simulink model "my_PUMA"  (Simulink 10.3)
settings: Solver=ode45  StartTime=0.0  StopTime=5  MaxStep=10  RelTol=1e-3  AbsTol=1e-6
StopFcn:
  | run('End_point_graph.m')
values from neighbouring files (symbols this model uses):
  k_p1 = (w_n1^2).*T_m1 ./ K1    [vars.m]
  k_p2 = (w_n2^2).*T_m2 ./ K2    [vars.m]
  k_p3 = (w_n3^2).*T_m3 ./ K3    [vars.m]
  k_v1 = 2*w_n1*zeta1*T_m1./(K1+1)    [vars.m]
  k_v2 = 2*w_n2*zeta2*T_m2./(K2+1)    [vars.m]
  k_v3 = 2*w_n3*zeta3*T_m3./(K3+1)    [vars.m]
  ng1 = 40+gn*4    [vars.m]
  ng2 = 100-gn*2    [vars.m]
  ng3 = 60+gn    [vars.m]
  thr10 = inital_angles(1)    [vars.m]
  thr20 = inital_angles(2)    [vars.m]
  thr30 = inital_angles(3)    [vars.m]
settings Model: Creator=Gu  LastModifiedBy=mubeen ak  MultithreadedSim=on
settings SolverCC: AutoScaleAbsTol=off
settings DataIOCC: SaveOutput=off  SaveTime=off  SignalLoggingName=sigsOut
settings OptimizationCC: BlockReduction=off  BooleanDataType=off  InitFltsAndDblsToZero=on
settings DebuggingCC: SaveWithParameterizedLinksMsg=none  SignalResolutionControl=TryResolveAllWithWarning  MultiTaskDSMMsg=warning  MultiTaskCondExecSysMsg=none  SFExecutionAtInitializationDiag=warning  SFMachineParentedDataDiag=error
settings HardwareCC: TargetUnknown=on
settings RTWCC: DLArmComputeVersion=20.02.1
settings GRTTargetCC: TargetFcnLib=ansi_tfl_tmw.mat
settings ConfigComp: CovSFcnEnable=off

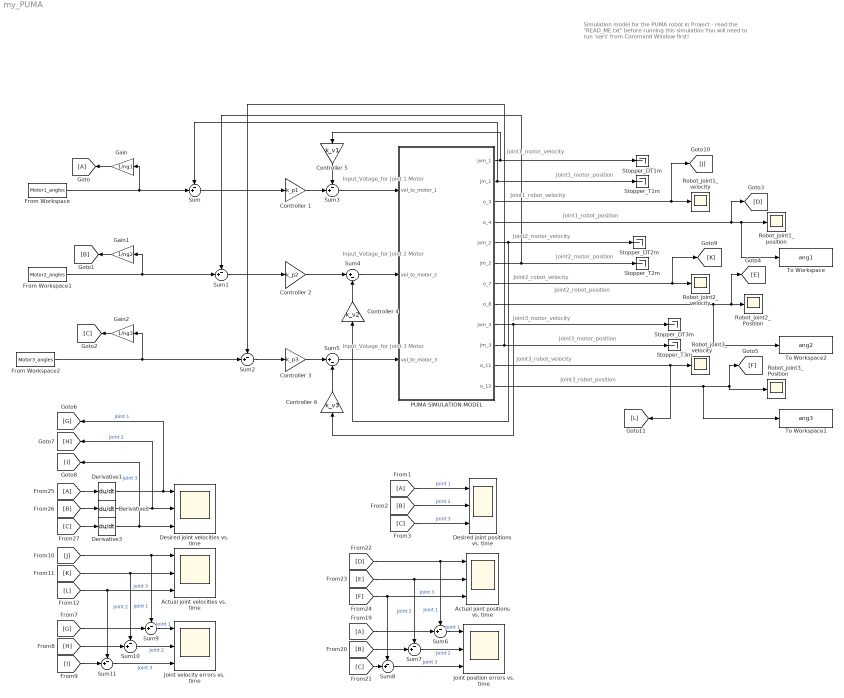
== system my_PUMA ==
  note: Joint1_motor_position
  note: Simulation model for the PUMA robot in Project - read the "READ_ME.txt" before running this simulation
      | You will need to run 'vars' from Command Window first!
  note: Joint2_motor_position
  note: Joint3_motor_position
  note: Joint1_motor_velocity
  note: Joint2_motor_velocity
  note: Joint3_motor_velocity
  note: Joint1_robot_velocity
  note: Joint2_robot_velocity
  note: Joint3_robot_velocity
  note: Joint1_robot_position
  note: Joint2_robot_position
  note: Joint3_robot_position
  note: Input_Votage_for Joint 3 Motor
  note: Input_Votage_for Joint 2 Motor
  note: Input_Votage_for Joint 1 Motor
  "Actual joint positions vs. time " : Scope  NumInputPorts=3
  "Actual joint velocities vs. time " : Scope  NumInputPorts=3
  Controller 1 : Gain  Gain=k_p1
  Controller 2 : Gain  Gain=k_p2
  Controller 3 : Gain  Gain=k_p3
  Controller 4 : Gain  Gain=k_v2
  Controller 5 : Gain  Gain=k_v1
  Controller 6 : Gain  Gain=k_v3
  Derivative1 : Derivative
  Derivative2 : Derivative
  Derivative3 : Derivative
  Desired joint positions vs. time : Scope  NumInputPorts=3
  "Desired joint velocities vs. time " : Scope  NumInputPorts=3
  From Workspace : FromWorkspace  VariableName=Motor1_angles  SampleTime=-1  OutputAfterFinalValue=Holding final value
  From Workspace1 : FromWorkspace  VariableName=Motor2_angles  OutDataTypeStr=double  SampleTime=-1  OutputAfterFinalValue=Holding final value
  From Workspace2 : FromWorkspace  VariableName=Motor3_angles  SampleTime=-1  OutputAfterFinalValue=Holding final value
  Gain : Gain  Gain=1/ng1
  Gain1 : Gain  Gain=1/ng2
  Gain2 : Gain  Gain=1/ng3
  Joint position errors vs. time : Scope  NumInputPorts=3
  "Joint velocity errors vs. time " : Scope  NumInputPorts=3
  PUMA SIMULATION MODEL : Subsystem
  Robot_joint1_position : Scope
  Robot_joint1_velocity : Scope
  Robot_joint2_Position : Scope
  Robot_joint2_velocity : Scope
  Robot_joint3_Position : Scope
  Robot_joint3_velocity : Scope
  Stopper_DT1m : Terminator
  Stopper_DT2m : Terminator
  Stopper_DT3m : Terminator
  Stopper_T1m : Terminator
  Stopper_T2m : Terminator
  Stopper_T3m : Terminator
  Sum{,1..3,6..11} (10 alike) : Sum  Inputs=-+|
  Sum4 : Sum  Inputs=|+-
  Sum5 : Sum  Inputs=|+-
  To Workspace : ToWorkspace  VariableName=ang1  SampleTime=-1
  To Workspace1 : ToWorkspace  VariableName=ang3  SampleTime=-1
  To Workspace2 : ToWorkspace  VariableName=ang2  SampleTime=-1
  wires:
  PUMA SIMULATION MODEL/4(o_4) -> [D], To Workspace/1, Robot_joint1_position/1
  PUMA SIMULATION MODEL/7(o_7) -> [K], Robot_joint2_velocity/1
  PUMA SIMULATION MODEL/8(o_8) -> To Workspace2/1, [E], Robot_joint2_Position/1
  PUMA SIMULATION MODEL/9(jvm_3) -> Controller 6/1, Stopper_DT3m/1
  PUMA SIMULATION MODEL/10(jm_3) -> Stopper_T3m/1, Sum2/1
  PUMA SIMULATION MODEL/12(o_12) -> To Workspace1/1, Robot_joint3_Position/1, [F]
  PUMA SIMULATION MODEL/2(jm_1) -> Stopper_T1m/1, Sum/1
  PUMA SIMULATION MODEL/6(jm_2) -> Stopper_T2m/1, Sum1/1
  PUMA SIMULATION MODEL/11(o_11) -> [L], Robot_joint3_velocity/1
  PUMA SIMULATION MODEL/3(o_3) -> [J], Robot_joint1_velocity/1
  Sum/1 -> Controller 1/1
  Sum1/1 -> Controller 2/1
  Controller 2/1 -> Sum4/1
  Controller 3/1 -> Sum5/1
  Sum2/1 -> Controller 3/1
  From Workspace1/1 -> Gain1/1, Sum1/2
  Sum3/1 -> PUMA SIMULATION MODEL/1(vol_to_motor_1)
  Controller 1/1 -> Sum3/2
  PUMA SIMULATION MODEL/1(jvm_1) -> Stopper_DT1m/1, Controller 5/1
  Sum4/1 -> PUMA SIMULATION MODEL/2(vol_to_motor_2)
  PUMA SIMULATION MODEL/5(jvm_2) -> Controller 4/1, Stopper_DT2m/1
  Controller 5/1 -> Sum3/1
  Controller 4/1 -> Sum4/2
  Controller 6/1 -> Sum5/2
  Sum5/1 -> PUMA SIMULATION MODEL/3(vol_to_motor_3)
  [A] -> Desired joint positions vs. time/1  "Joint 1"
  [B] -> Desired joint positions vs. time/2  "Joint 2"
  [C] -> Desired joint positions vs. time/3  "Joint 3"
  [L] -> Sum11/1, "Actual joint velocities vs. time "/3  "Joint 3"
  [J] -> Sum9/1, "Actual joint velocities vs. time "/1  "Joint 1"
  [K] -> Sum10/1, "Actual joint velocities vs. time "/2  "Joint 2"
  Gain/1 -> [A]
  Gain1/1 -> [B]
  Gain2/1 -> [C]
  Sum6/1 -> Joint position errors vs. time/1  "Joint 1"
  [C] -> Sum8/2
  [B] -> Sum7/2
  [A] -> Sum6/2
  Sum7/1 -> Joint position errors vs. time/2  "Joint 2"
  Sum8/1 -> Joint position errors vs. time/3  "joint 3"
  [D] -> "Actual joint positions vs. time "/1, Sum6/1  "Joint 1"
  [E] -> "Actual joint positions vs. time "/2, Sum7/1  "Joint 2"
  [F] -> "Actual joint positions vs. time "/3, Sum8/1  "Joint 3"
  [A] -> Derivative1/1
  [B] -> Derivative2/1
  [C] -> Derivative3/1
  Derivative1/1 -> [G], "Desired joint velocities vs. time "/1  "Joint 1"
  Derivative2/1 -> [H], "Desired joint velocities vs. time "/2  "Joint 2"
  Derivative3/1 -> [I], "Desired joint velocities vs. time "/3  "Joint 3"
  Sum9/1 -> "Joint velocity errors vs. time "/1  "Joint 1"
  Sum10/1 -> "Joint velocity errors vs. time "/2  "Joint 2"
  Sum11/1 -> "Joint velocity errors vs. time "/3  "Joint 3"
  [G] -> Sum9/2
  [H] -> Sum10/2
  [I] -> Sum11/2
  From Workspace2/1 -> Sum2/2, Gain2/1
  From Workspace/1 -> Gain/1, Sum/2

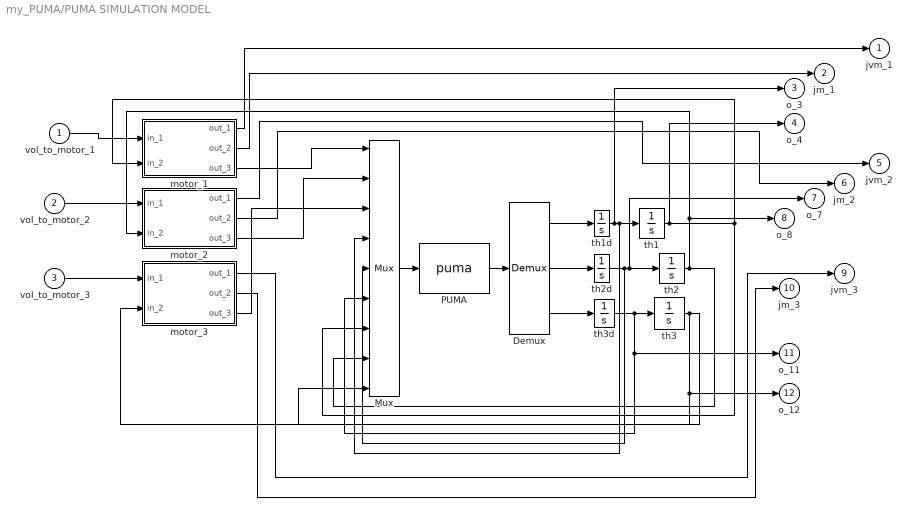
== system my_PUMA/PUMA SIMULATION MODEL ==
  vol_to_motor_1 : Inport
  vol_to_motor_2 : Inport  Port=2
  vol_to_motor_3 : Inport  Port=3
  Demux : Demux  Outputs=3
      settings: DisplayOption=none
  Mux : Mux  Inputs=9
  PUMA : MATLABFcn  MATLABFcn=puma  OutputDimensions=3
  motor_1 : Subsystem
  motor_2 : Subsystem
  motor_3 : Subsystem
  th1 : Integrator  InitialCondition=thr10
  th1d : Integrator
  th2 : Integrator  InitialCondition=thr20
  th2d : Integrator
  th3 : Integrator  InitialCondition=thr30
  th3d : Integrator
  jvm_1 : Outport  InitialOutput=0  VectorParamsAs1DForOutWhenUnconnected=off
  jm_1 : Outport  Port=2  InitialOutput=0  VectorParamsAs1DForOutWhenUnconnected=off
  o_3 : Outport  Port=3  InitialOutput=0  VectorParamsAs1DForOutWhenUnconnected=off
  o_4 : Outport  Port=4  InitialOutput=0  VectorParamsAs1DForOutWhenUnconnected=off
  jvm_2 : Outport  Port=5  InitialOutput=0  VectorParamsAs1DForOutWhenUnconnected=off
  jm_2 : Outport  Port=6  InitialOutput=0  VectorParamsAs1DForOutWhenUnconnected=off
  o_7 : Outport  Port=7  InitialOutput=0  VectorParamsAs1DForOutWhenUnconnected=off
  o_8 : Outport  Port=8  InitialOutput=0  VectorParamsAs1DForOutWhenUnconnected=off
  jvm_3 : Outport  Port=9  InitialOutput=0  VectorParamsAs1DForOutWhenUnconnected=off
  jm_3 : Outport  Port=10  InitialOutput=0  VectorParamsAs1DForOutWhenUnconnected=off
  o_11 : Outport  Port=11  InitialOutput=0  VectorParamsAs1DForOutWhenUnconnected=off
  o_12 : Outport  Port=12  InitialOutput=0  VectorParamsAs1DForOutWhenUnconnected=off
  wires:
  motor_3/2(out_2) -> jm_3/1
  motor_3/1(out_1) -> jvm_3/1
  motor_2/2(out_2) -> jm_2/1
  motor_2/1(out_1) -> jvm_2/1
  motor_1/2(out_2) -> jm_1/1
  motor_1/1(out_1) -> jvm_1/1
  vol_to_motor_2/1 -> motor_2/1(in_1)
  motor_3/3(out_3) -> Mux/3
  motor_2/3(out_3) -> Mux/2
  motor_1/3(out_3) -> Mux/1
  vol_to_motor_3/1 -> motor_3/1(in_1)
  vol_to_motor_1/1 -> motor_1/1(in_1)
  th3d/1 -> Mux/6, o_11/1, th3/1
  th2d/1 -> Mux/5, o_7/1, th2/1
  PUMA/1 -> Demux/1
  th2/1 -> Mux/8, o_8/1, motor_2/2(in_2)
  th1/1 -> Mux/7, motor_1/2(in_2), o_4/1
  th3/1 -> Mux/9, o_12/1, motor_3/2(in_2)
  th1d/1 -> Mux/4, th1/1, o_3/1
  Demux/3 -> th3d/1
  Demux/2 -> th2d/1
  Demux/1 -> th1d/1
  Mux/1 -> PUMA/1

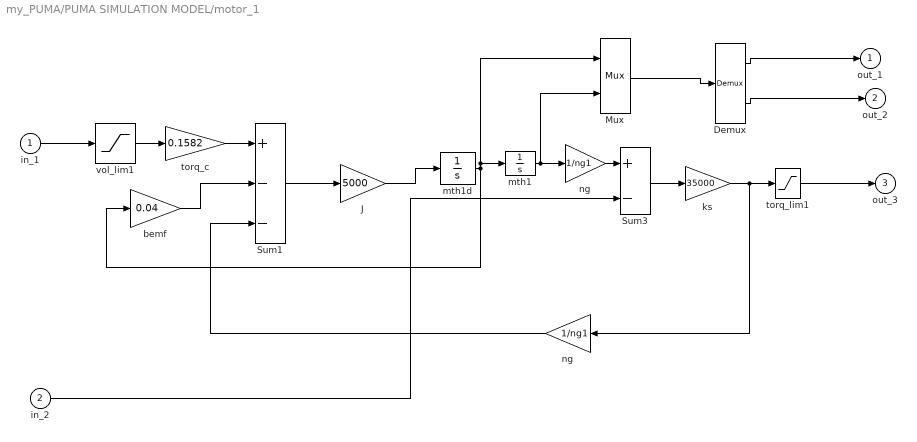
== system my_PUMA/PUMA SIMULATION MODEL/motor_1 ==
  in_1 : Inport
  in_2 : Inport  Port=2
  Demux : Demux  Outputs=2
      settings: DisplayOption=none
  J : Gain  Gain=5000  SaturateOnIntegerOverflow=on  OutDataTypeStr=Inherit: Same as input  ParamDataTypeStr=Inherit: Same as input
  Mux : Mux  Inputs=2
  Sum1 : Sum  Inputs=+--  InputSameDT=on  SaturateOnIntegerOverflow=on  OutDataTypeStr=Inherit: Same as first input
  Sum3 : Sum  Inputs=+-  InputSameDT=on  SaturateOnIntegerOverflow=on  OutDataTypeStr=Inherit: Same as first input
  bemf : Gain  Gain=0.04  SaturateOnIntegerOverflow=on  OutDataTypeStr=Inherit: Same as input  ParamDataTypeStr=Inherit: Same as input
  ks : Gain  Gain=35000  SaturateOnIntegerOverflow=on  OutDataTypeStr=Inherit: Same as input  ParamDataTypeStr=Inherit: Same as input
  mth1 : Integrator  InitialCondition=ng1*thr10
  mth1d : Integrator
  ng : Gain  Gain=1/ng1  SaturateOnIntegerOverflow=on  OutDataTypeStr=Inherit: Same as input  ParamDataTypeStr=Inherit: Same as input
  "ng " : Gain  Gain=1/ng1  SaturateOnIntegerOverflow=on  OutDataTypeStr=Inherit: Same as input  ParamDataTypeStr=Inherit: Same as input
  torq_c : Gain  Gain=0.1582  SaturateOnIntegerOverflow=on  OutDataTypeStr=Inherit: Same as input  ParamDataTypeStr=Inherit: Same as input
  torq_lim1 : Saturate  UpperLimit=1.2*ng1  LowerLimit=-1.2*ng1
  vol_lim1 : Saturate  UpperLimit=40  LowerLimit=-40
  out_1 : Outport  InitialOutput=0  VectorParamsAs1DForOutWhenUnconnected=off
  out_2 : Outport  Port=2  InitialOutput=0  VectorParamsAs1DForOutWhenUnconnected=off
  out_3 : Outport  Port=3  InitialOutput=0  VectorParamsAs1DForOutWhenUnconnected=off
  wires:
  in_2/1 -> Sum3/2
  bemf/1 -> Sum1/2
  J/1 -> mth1d/1
  Sum1/1 -> J/1
  "ng "/1 -> Sum1/3
  ng/1 -> Sum3/1
  Sum3/1 -> ks/1
  mth1d/1 -> mth1/1, Mux/1, bemf/1
  torq_c/1 -> Sum1/1
  vol_lim1/1 -> torq_c/1
  in_1/1 -> vol_lim1/1
  torq_lim1/1 -> out_3/1
  ks/1 -> "ng "/1, torq_lim1/1
  mth1/1 -> Mux/2, ng/1
  Mux/1 -> Demux/1
  Demux/1 -> out_1/1
  Demux/2 -> out_2/1

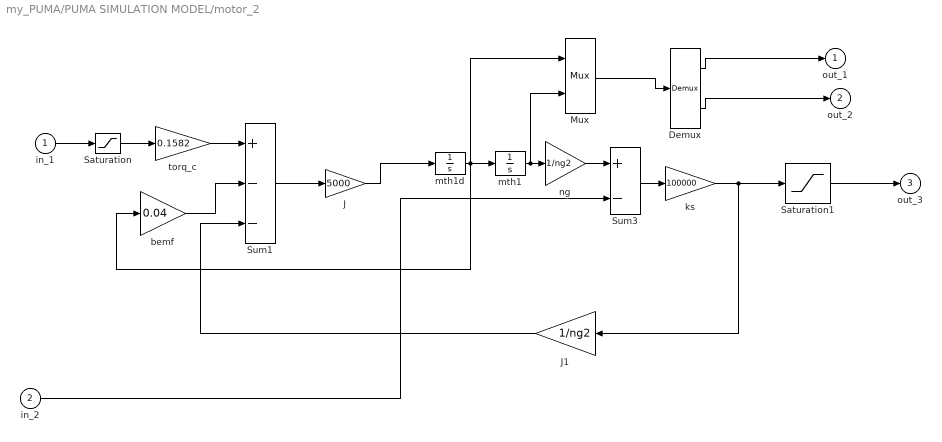
== system my_PUMA/PUMA SIMULATION MODEL/motor_2 ==
  in_1 : Inport
  in_2 : Inport  Port=2
  Demux : Demux  Outputs=2
      settings: DisplayOption=none
  J : Gain  Gain=5000  SaturateOnIntegerOverflow=on  OutDataTypeStr=Inherit: Same as input  ParamDataTypeStr=Inherit: Same as input
  J1 : Gain  Gain=1/ng2  SaturateOnIntegerOverflow=on  OutDataTypeStr=Inherit: Same as input  ParamDataTypeStr=Inherit: Same as input
  Mux : Mux  Inputs=2
  Saturation : Saturate  UpperLimit=40  LowerLimit=-40
  Saturation1 : Saturate  UpperLimit=ng2*1.2  LowerLimit=-ng2*1.2
  Sum1 : Sum  Inputs=+--  InputSameDT=on  SaturateOnIntegerOverflow=on  OutDataTypeStr=Inherit: Same as first input
  Sum3 : Sum  Inputs=+-  InputSameDT=on  SaturateOnIntegerOverflow=on  OutDataTypeStr=Inherit: Same as first input
  bemf : Gain  Gain=0.04  SaturateOnIntegerOverflow=on  OutDataTypeStr=Inherit: Same as input  ParamDataTypeStr=Inherit: Same as input
  ks : Gain  Gain=100000  SaturateOnIntegerOverflow=on  OutDataTypeStr=Inherit: Same as input  ParamDataTypeStr=Inherit: Same as input
  mth1 : Integrator  InitialCondition=thr20*ng2
  mth1d : Integrator
  ng : Gain  Gain=1/ng2  SaturateOnIntegerOverflow=on  OutDataTypeStr=Inherit: Same as input  ParamDataTypeStr=Inherit: Same as input
  torq_c : Gain  Gain=0.1582  SaturateOnIntegerOverflow=on  OutDataTypeStr=Inherit: Same as input  ParamDataTypeStr=Inherit: Same as input
  out_1 : Outport  InitialOutput=0  VectorParamsAs1DForOutWhenUnconnected=off
  out_2 : Outport  Port=2  InitialOutput=0  VectorParamsAs1DForOutWhenUnconnected=off
  out_3 : Outport  Port=3  InitialOutput=0  VectorParamsAs1DForOutWhenUnconnected=off
  wires:
  in_2/1 -> Sum3/2
  bemf/1 -> Sum1/2
  J/1 -> mth1d/1
  Sum1/1 -> J/1
  J1/1 -> Sum1/3
  ng/1 -> Sum3/1
  Sum3/1 -> ks/1
  mth1d/1 -> bemf/1, mth1/1, Mux/1
  torq_c/1 -> Sum1/1
  Saturation/1 -> torq_c/1
  in_1/1 -> Saturation/1
  ks/1 -> J1/1, Saturation1/1
  Saturation1/1 -> out_3/1
  Mux/1 -> Demux/1
  mth1/1 -> Mux/2, ng/1
  Demux/1 -> out_1/1
  Demux/2 -> out_2/1

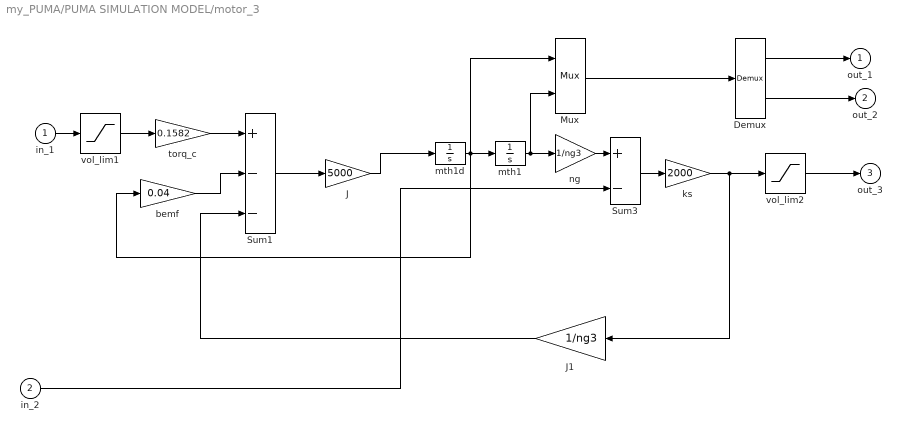
== system my_PUMA/PUMA SIMULATION MODEL/motor_3 ==
  in_1 : Inport
  in_2 : Inport  Port=2
  Demux : Demux  Outputs=2
      settings: DisplayOption=none
  J : Gain  Gain=5000  SaturateOnIntegerOverflow=on  OutDataTypeStr=Inherit: Same as input  ParamDataTypeStr=Inherit: Same as input
  J1 : Gain  Gain=1/ng3  SaturateOnIntegerOverflow=on  OutDataTypeStr=Inherit: Same as input  ParamDataTypeStr=Inherit: Same as input
  Mux : Mux  Inputs=2
  Sum1 : Sum  Inputs=+--  InputSameDT=on  SaturateOnIntegerOverflow=on  OutDataTypeStr=Inherit: Same as first input
  Sum3 : Sum  Inputs=+-  InputSameDT=on  SaturateOnIntegerOverflow=on  OutDataTypeStr=Inherit: Same as first input
  bemf : Gain  Gain=0.04  SaturateOnIntegerOverflow=on  OutDataTypeStr=Inherit: Same as input  ParamDataTypeStr=Inherit: Same as input
  ks : Gain  Gain=2000  SaturateOnIntegerOverflow=on  OutDataTypeStr=Inherit: Same as input  ParamDataTypeStr=Inherit: Same as input
  mth1 : Integrator  InitialCondition=thr30*ng3
  mth1d : Integrator
  ng : Gain  Gain=1/ng3  SaturateOnIntegerOverflow=on  OutDataTypeStr=Inherit: Same as input  ParamDataTypeStr=Inherit: Same as input
  torq_c : Gain  Gain=0.1582  SaturateOnIntegerOverflow=on  OutDataTypeStr=Inherit: Same as input  ParamDataTypeStr=Inherit: Same as input
  vol_lim1 : Saturate  UpperLimit=40  LowerLimit=-40
  vol_lim2 : Saturate  UpperLimit=1.2*ng3  LowerLimit=-1.2*ng3
  out_1 : Outport  InitialOutput=0  VectorParamsAs1DForOutWhenUnconnected=off
  out_2 : Outport  Port=2  InitialOutput=0  VectorParamsAs1DForOutWhenUnconnected=off
  out_3 : Outport  Port=3  InitialOutput=0  VectorParamsAs1DForOutWhenUnconnected=off
  wires:
  in_2/1 -> Sum3/2
  bemf/1 -> Sum1/2
  J/1 -> mth1d/1
  Sum1/1 -> J/1
  J1/1 -> Sum1/3
  ng/1 -> Sum3/1
  Sum3/1 -> ks/1
  mth1d/1 -> bemf/1, mth1/1, Mux/1
  torq_c/1 -> Sum1/1
  Mux/1 -> Demux/1
  mth1/1 -> Mux/2, ng/1
  vol_lim1/1 -> torq_c/1
  in_1/1 -> vol_lim1/1
  vol_lim2/1 -> out_3/1
  ks/1 -> J1/1, vol_lim2/1
  Demux/1 -> out_1/1
  Demux/2 -> out_2/1
